simulink model "Torque_Vectoring_Controller_dSpace_RTI1401"  (R2016a)
settings: Solver=ode1  StartTime=0.0  StopTime=Inf  FixedStep=car.dt  RelTol=1e-3
PostLoadFcn:
  | , if any(exist('dsrtsu_mdlpostloadfcn', 'file') == [2, 3, 6]), try dsrtsu_mdlpostloadfcn('Execute', bdroot); catch fprintf('Error in PostLoadFcn (dsrtsu_mdlpostloadfcn) for model "%s":\n %s\n', bdroot, lasterr); end, end,
InitFcn:
  | clear_close
  | dataCar
  | optParam
  | structSensors
  | structSettings
  | structEstimPar
  | structAero
  | structVariables
  | readFuzzyFile
StartFcn:
  | clear_close
  | dataCar
  | optParam
  | structSensors
  | structSettings
  | structEstimPar
  | structAero
  | structVariables
  | readFuzzyFile
undefined symbols (not defined in the file or in its folder): car, optPar
libraries: fuzblock x1
(part 2 of 2)

== matlab function Torque_Vectoring_Controller_dSpace_RTI1401/Controls/Vehicle Estimated Parameters/Velocity Estimator/Velicity Estimator 2 ==
  data: sensors input; v2 output; settings input; car parameter; vCOG output
function [v2,vCOG] = Velocity_Estimator1(sensors, settings,  car)

vycog = 0;
dist = [car.lf car.lf -car.lr -car.lr;
  car.tw/2 -car.tw/2 car.tw/2 -car.tw/2;
  0 0 0 0];
wheelAngle = (sensors.wheelAngles(1)+sensors.wheelAngles(2))/2;

%tw_dist = [-car.tw/2 car.tw/2 -car.tw/2 car.tw/2];
      

% Note: axis systems X,Y,Z in car frame, x,y,z in wheel frame.
%X:forward
%Y:left
%Z:up


RxyzXYZ=[cos(wheelAngle) sin(wheelAngle) 0;
   -sin(wheelAngle) cos(wheelAngle) 0;
   0 0 1];
omega = [0 0 0 0 ;
   sensors.wheelspeed(1) sensors.wheelspeed(2) sensors.wheelspeed(3) sensors.wheelspeed(4)
   ;0 0 0 0];
radius = [0;0;-car.tireRadius];
yawRate = [0;0;sensors.yawRate];

% wheelspeed = [sensors.wheelspeed(1) sensors.wheelspeed(2) sensors.wheelspeed(3) sensors.wheelspeed(4)];
% steeringAngle = [wheelAngle;wheelAngle;0;0];
% omegaR = [sensors.wheelspeed(1); sensors.wheelspeed(2); sensors.wheelspeed(3); sensors.wheelspeed(4)].*car.tireRadius;


% persistent vCOG_m
% if isempty(vCOG_m); vCOG_m = zeros(3,4); end

% persistent vxCOG
% if isempty(vxCOG); vxCOG = zeros(4,1); end
vCOG_m = zeros(3,4);
vCOG = zeros(4,1);

%vxCOG_m = zeros(4,1);


%Can be faster without the matrices
%Slip can be taken into account by v_wheel(now=0,changing it to velocity with slip) =
%RxyzXYZ*cross(wheelspeed,tireRadius)+cross(yawRate,dist)+vXYZ
 
for i=1:4
    vCOG_m(:,i) = -(RxyzXYZ*cross(omega(:,i),radius)+cross(yawRate,dist(:,i)));  %%SteeringAngle is not yet changed for the rear wheels w
    vCOG(i,1) = sqrt(vCOG_m(1,i)^2+vCOG_m(2,i)^2);
    %vxCOG_m(i,1)=vCOG_m(1,i);
    %vxCOG(i,1)=-(cos(steeringAngle(i))*(car.tireRadius*wheelspeed(i))-sensors.yawRate*tw_dist(i));
end

% Select/average based on wheel speed
axtol = 2; % Tolerance to detect acceleration / deceleration [m/s2]
if sensors.ax > axtol
    vEst_wheels = min(vCOG);    %lowest wheelspeed to take possible slip into account
elseif sensors.ax < -axtol
    vEst_wheels = max(vCOG);    %highest wheelspeed to take possible wheel lock into account
else
    vEst_wheels = median(vCOG); % Note: median is less sensitive to outliers
end




v2= vEst_wheels;

== matlab function Torque_Vectoring_Controller_dSpace_RTI1401/Controls/Vehicle Estimated Parameters/Velocity Estimator/Velocity_Estimator3 ==
  data: sensors input; v3 output; settings input; car parameter; v input
function v3  = Velocity_Estimator3(sensors, settings,  car, v)

persistent vActual; if isempty(vActual); vActual = 0; end


%IMPORTANT: change car.fECU and car.dt when changing operating speed in Simulink

v3 = vActual + sensors.ax * car.dt;

vActual = v;

== matlab function Torque_Vectoring_Controller_dSpace_RTI1401/Controls/Vehicle Estimated Parameters/Velocity Estimator/MATLAB Function ==
  data: v output; vFuzzy input
function v = fcn(vFuzzy)
%#codegen

v = vFuzzy;

== matlab function Torque_Vectoring_Controller_dSpace_RTI1401/Controls/Vehicle Estimated Parameters/Velocity Estimator/Kalman Velocity ==
  data: sensors input; settings input; v2 input; vKalman output; v4 input; car parameter
function vKalman = Velocity_EstimatorKalman(sensors,settings,v2,v4,car)


% Keep track of the estimated velocity
persistent vEst; if isempty(vEst); vEst = 0; end;
persistent PEst; if isempty(PEst); PEst = 0; end;

% Model
A = 1; B = car.dt;
H = [1;1];
Q = car.kalmanVelocity.Q;
R = car.kalmanVelocity.R;

% Measurements
y = [v2; v4];

% if settings.velocityEstimation == 0 || settings.velocityEstimation == 1 || vEst < car.speed.velTreshold || sensors.vboxX < car.speed.velTreshold
%     %vbox disabled
%     H(1) = 0;
% end



% === Time update ===
vEst = A*vEst + B*sensors.ax;
PEst = A*PEst*A' + Q;

% === Measurement update ===
K = PEst*H'/(H*PEst*H'+R);
vEst = vEst + K*(y-H*vEst);
PEst = (1-K*H)*PEst;
% Output
vest_out = vEst;

%sensors_out = sensors;
%sensors_out.vx = vest_out;
vKalman = vest_out;

== matlab function Torque_Vectoring_Controller_dSpace_RTI1401/Controls/Vehicle Estimated Parameters/Velocity Estimator/Fuzzy Velocity/FuzzyVelicityGenerator ==
  data: k1 input; vFuzzy output; k2 input; k3 input; k4 input; k5 input; sensors input; settings input; car parameter
function vFuzzy = fuzzyVelocityGenerator(k1,k2,k3,k4,k5,sensors,settings,car)

persistent vFuzzyPrev; if isempty(vFuzzyPrev); vFuzzyPrev = 0; end

beta=0;


vRFL_COG = (sensors.wheelspeed(1)*car.tireRadius...
    + sensors.yawRate*(car.tw/2-car.lf*beta))...
    *cos(sensors.wheelAngles(1)-beta);
vRFR_COG = (sensors.wheelspeed(2)*car.tireRadius...
    - sensors.yawRate*(car.tw/2+car.lf*beta))...
    *cos(sensors.wheelAngles(2)-beta);
vRRL_COG = (sensors.wheelspeed(3)*car.tireRadius...
    + sensors.yawRate*(car.tw/2+car.lr*beta))...
    *cos(beta);
vRRR_COG = (sensors.wheelspeed(4)*car.tireRadius...
    - sensors.yawRate*(car.tw/2-car.lr*beta))...
    *cos(beta);
vR_COG=[vRFL_COG;vRFR_COG;vRRL_COG;vRRR_COG];

vFuzzy = (sum([k1;k2;k3;k4].*vR_COG)+k5*(vFuzzyPrev+car.dt*sensors.ax))...
    /(k1+k2+k3+k4+k5);

vFuzzyPrev = vFuzzy;

== matlab function Torque_Vectoring_Controller_dSpace_RTI1401/Controls/Vehicle Estimated Parameters/Velocity Estimator/Fuzzy Velocity/fuzzyParam ==
  data: sensors input; deltaVFL output; settings input; vFuzzyPrev input; deltaVFR output; deltaVRL output; deltaVRR output; maxDeltaV output; car parameter
function [deltaVFL,deltaVFR,deltaVRL,deltaVRR,maxDeltaV]= fuzzyParam(sensors, settings,vFuzzyPrev,car)
beta=0;
vRFL_COG = (sensors.wheelspeed(1)*car.tireRadius...
    + sensors.yawRate*(car.tw/2-car.lf*beta))...
    *cos(sensors.wheelAngles(1)-beta);
vRFR_COG = (sensors.wheelspeed(2)*car.tireRadius...
    - sensors.yawRate*(car.tw/2+car.lf*beta))...
    *cos(sensors.wheelAngles(2)-beta);
vRRL_COG = (sensors.wheelspeed(3)*car.tireRadius...
    + sensors.yawRate*(car.tw/2+car.lr*beta))...
    *cos(beta);
vRRR_COG = (sensors.wheelspeed(4)*car.tireRadius...
    - sensors.yawRate*(car.tw/2-car.lr*beta))...
    *cos(beta);
vR_COG=[vRFL_COG;vRFR_COG;vRRL_COG;vRRR_COG];

deltaVFL = vRFL_COG-vFuzzyPrev;
deltaVFR = vRFR_COG-vFuzzyPrev;
deltaVRL = vRRL_COG-vFuzzyPrev;
deltaVRR = vRRR_COG-vFuzzyPrev;

maxDeltaV = abs(vFuzzyPrev-max(vR_COG))+abs(vFuzzyPrev-min(vR_COG));

== matlab function Torque_Vectoring_Controller_dSpace_RTI1401/Controls/Subsystem/MATLAB Function ==
  data: torqueController input; torques output; rpmController input; torqueBypass input; rpmBypass input; rpmRef output; settings input
function [torques,rpmRef]= fcn(torqueController,rpmController,torqueBypass,rpmBypass,settings)
%#codegen

torques = [0;0;0;0];
rpmRef = [0;0;0;0];

if settings.TV_bypass == 0

    torques = torqueController;
    rpmRef = rpmController;

elseif settings.TV_bypass == 1
    
    torques = torqueBypass;
    rpmRef = rpmBypass;
end

== matlab function Torque_Vectoring_Controller_dSpace_RTI1401/Controls/Control Systems/Distributor/Torque//Brake analyzer/MATLAB Function1 ==
  data: sensors input; Fdes output; settings input; estimPar input; variables input; car parameter
function Fdes = Fdes(sensors, settings, estimPar, variables,car)
    


%Fdes = 11*4* min(car.motor.Tmax)*variables.TD_percentage*sensors.throttle/car.tireRadius;
    %if sensors.throttle > 0
    %Fdes = sum(car.motor.Tmax)*variables.TD_percentage*sensors.throttle/car.tireRadius; % *4 because four motors
    %Fdes = Fdes*car.gearRatio;
    
    Fdes = sum(sensors.throttle*1.5*estimPar.mu*(car.mass*car.g + 0.5*car.rhoAir*estimPar.v*estimPar.v*car.Cl*car.AFront));
    
    if sensors.brake > 0
        Fdes = -sum(car.motor.Tmax)*variables.TD_percentage*sensors.brake/car.tireRadius;
        Fdes = Fdes*car.gearRatio;
    end
    %Fdes= 5000;
    
    %end
    %     Fdes = Fdes*1;
    %     Fdes = 800;
    
    %     Fdes = sensors.throttle*mean(estimPar.mu)*(car.mass*car.g + 0.5*car.rhoAir*estimPar.v*estimPar.v*car.Cl*car.AFront );
    %     Fdes = Fdes;
    

end

== matlab function Torque_Vectoring_Controller_dSpace_RTI1401/Controls/Control Systems/Power Checker/Power checker ==
  data: sensors input; settings input; estimPar input; UncheckedTorque input; CheckedTorque output; car parameter; P_mech output; maxMechPower output; power2beReduced output; part2beReduced output; CheckedP_mech output
function [CheckedTorque,P_mech,maxMechPower,power2beReduced,part2beReduced,CheckedP_mech]= fcn(sensors, settings,estimPar, UncheckedTorque, car)

%% Power limiter according to FS rules

P_mech = sum(UncheckedTorque.*sensors.wheelspeed*car.gearRatio); %[Nm*rad/s][W]

maxMechPower = (car.Pmax - car.PC.safetyMargin)*estimPar.eff;
power2beReduced = 0;

if P_mech > maxMechPower
    power2beReduced = P_mech - maxMechPower;
end

if abs(P_mech) > 0.1
    part2beReduced = power2beReduced/P_mech;
else
    part2beReduced = 0;
end

CheckedTorque = UncheckedTorque*max(min((1 - part2beReduced),1),0);
CheckedP_mech = sum(CheckedTorque.*sensors.wheelspeed*car.gearRatio); %[Nm*rad/s][W]

== matlab function Torque_Vectoring_Controller_dSpace_RTI1401/Controls/Vehicle Estimated Parameters/Efficiency Estimator ==
  data: sensors input; eff output; settings input; car parameter; P_elec output; P_mech output; effnotcontrolled output
function [eff,P_elec,P_mech,effnotcontrolled]= Efficiency(sensors,settings,car)
%P_elec * eff = P_mech

persistent effTemp; if isempty(effTemp); effTemp = 0.7; end
persistent errorInt; if isempty(errorInt); errorInt = 0; end

Pmax = car.Pmax - car.PC.safetyMargin; %[W]

P_mech = sum(sensors.torque.*sensors.wheelspeed); %*car.gearRatio
P_elec = sensors.P_elec;
ratio = 0.2;

if settings.effEstimation == 1
    
    if P_elec > 1
        effCalc = P_mech/P_elec;
        effTemp = effTemp*ratio + (1-ratio)*min(max(effCalc,car.PC.minEff),car.PC.maxEff);
        
    elseif P_elec < 1
        effCalc = P_elec/min(P_mech,-1);
        effTemp = effTemp*ratio + (1-ratio)*min(max(effCalc,car.PC.minEff),car.PC.maxEff);
        
        
        %mogelijkheid tot uitbreiding: Pmax variable ifv van batterij voor tijdens
        %indurance
    end
    
end

if settings.effEstimation == 2
    
    if P_elec > Pmax*0.3 && sensors.throttle > 0 % only positive power limit
        
        error = (Pmax - P_elec)/Pmax;
        if error < 0 % P_elec > Pmax
            error = error*2;
        end
        
        errorInt = errorInt + error*car.dt;
        errorInt = max(min(errorInt,0.2),-0.2);
        
        dEff = car.PC.Kp*error + car.PC.Ki*errorInt; %more fitting variable name would be powerReductionFactor as this is not anymore an efficiency as Pelec * eff = Pmech
        %make car.PC.Kp velocity dependend?
        
        effTemp = max(min(effTemp + dEff,car.PC.maxEff),car.PC.minEff);
        
    else
        if P_elec > 5000
            eta = P_mech/P_elec;
            effTemp = effTemp*ratio+(1-ratio)*min(max(eta,car.PC.minEff),car.PC.maxEff);
        elseif P_elec < -5000
            eta = P_elec/min(P_mech,-1);
            effTemp = effTemp*ratio+(1-ratio)*min(max(eta,car.PC.minEff),car.PC.maxEff);
        end
        
    end
    
else
    effTemp = effTemp;
    
end


eff = effTemp;
effnotcontrolled = P_mech/P_elec;

== matlab function Torque_Vectoring_Controller_dSpace_RTI1401/Controls/Vehicle Estimated Parameters/Yaw Rate Reference ==
  data: sensors input; rref output; settings input; v input; car parameter
function rref = yawRateRef(sensors, settings, v, car)
if isempty(v); v =0;end
%Ackermann
wheelAngle = (sensors.wheelAngles(1)+sensors.wheelAngles(2))/2;
rref = wheelAngle*v/car.wb;




% 
% des_yaw_rate = vx*steering_angle / ...
%     (L_f + L_r + ...
%     m_chassis*vx^2*(L_r*(C_x_alpha_RL+C_x_alpha_RR)-L_f*(C_x_alpha_FL+C_x_alpha_FR))/...
%     ((C_x_alpha_RL+C_x_alpha_RR)*(C_x_alpha_FL+C_x_alpha_FR)*L));

== matlab function Torque_Vectoring_Controller_dSpace_RTI1401/Vehicle Sensors/Sensors ==
  data: ax input; sensors output Bus: sensorBus size=1; ay input; wheelspeed_FL input; wheelspeed_FR input; wheelspeed_RL input; wheelspeed_RR input; yawRate input; steeringAngle input; steerAngleFL input; steerAngleFR input; throttle input; brake input; torqueFL input; torqueFR input; torqueRL input; torqueRR input; ax_error input; ay_error input; yawRate_error input; knob1 input; knob2 input; P_elec_FL input; P_elec_FR input; P_elec_RL input; P_elec_RR input
function sensors = sensors(ax,ay,wheelspeed_FL,wheelspeed_FR,wheelspeed_RL,wheelspeed_RR,yawRate,steeringAngle,steerAngleFL,steerAngleFR, throttle,brake,torqueFL,torqueFR,torqueRL,torqueRR,ax_error,ay_error,yawRate_error,knob1,knob2,P_elec_FL,P_elec_FR,P_elec_RL,P_elec_RR)

sensors.ax = ax;
sensors.ay = ay;
sensors.wheelspeed = [wheelspeed_FL;wheelspeed_FR;wheelspeed_RL;wheelspeed_RR];
sensors.yawRate = yawRate;
sensors.steerAngle = steeringAngle;
sensors.wheelAngles = [steerAngleFL;steerAngleFR;0;0];
sensors.throttle = throttle;
sensors.brake= brake;
sensors.torque = [torqueFL;torqueFR;torqueRL;torqueRR];
sensors.ax_error = ax_error;
sensors.ay_error = ay_error;
sensors.yawRate_error = yawRate_error;
sensors.knob1 = knob1;
sensors.knob2 = knob2;
sensors.P_elec = sum([P_elec_FL;P_elec_FR;P_elec_RL;P_elec_RR]);
